simulink model "part2_MAIN_2019_for_ayon_because_he_cant_update_his_matlab"  (R2019a)
settings: Solver=FixedStepAuto  StartTime=0.0  StopTime=300  FixedStep=0.1  RelTol=1e-3
values from neighbouring files (symbols this model uses):
  Af = diag(ti)    [init.m]    (also in init_old.m)
  Aw = [zeros(3) eye(3) ... (first row only)    [get_observer_parameters.m]
  B = [thr1 thr2_x thr2_y thr3 thr4_x thr4_y thr5_x thr5_y]    [B_redistributed.m]    (also in check_alg.m = [1 2 3 4 5 6 7 8; get_observer_parameters.m = [zeros(6,3);zeros(3,3);zeros(3,3);inv(M)])
  change_position_time = 1200    [init.m]    (also in init_old.m)
  Cw = [zeros(3) eye(3)]    [get_observer_parameters.m]
  D = Damping    [init.m]    (also in init_old.m)
  Damping = diag([2.6486e5, 8.8164e5, 3.3774e8])    [init.m]    (also in init_old.m)
  direction_limit = pi/36    (= 0.0872664625997)    [init.m]    (also in init_old.m)
  direction_time_constant = 100    [init.m]    (also in init_old.m)
  dt = 0.1    [get_observer_parameters.m]
  E = [Ew, zeros(6,3) ... (first row only)    [get_observer_parameters.m]
  Gamma = diag(omega_is)    [init.m]    (also in init_old.m)
  gust_limit = 40    [init.m]    (also in init_old.m)
  H = [Cw, eye(3), zeros(3,3) zeros(3,3)]    [get_observer_parameters.m]    (also in quadprog.m = 2*diag([w.' w.' q.' q.' w_alpha.' w_alpha.']); quadprog_basic.m = 2*diag([w.' w.' q.' q.']); quadprog_false.m = 2*diag([w.' w.' q.' q.' w_alpha.' w_alpha.']))
  height = 3    [init.m]    (also in init_old.m)
  inv_M = inv(M)    [get_observer_parameters.m]
  inv_Tb = inv(Tb)    [get_observer_parameters.m]
  kappa = 0.003    [init.m]    (also in init_old.m)
  kappa2 = 0.0026    [init.m]    (also in init_old.m)
  Kd = [1660451.40544401; 3920391.80535684; 1605063439.04156]    [init.m]    (also in init_old.m)
  Ki = [137.081306245593; 3163.274947400198; 335358.448218978]    [init.m]    (also in init_old.m)
  Kp = [75459.3345349083; 277551.73586971; 120744473.878042]    [init.m]    (also in init_old.m)
  L = 1800    [init.m]    (also in init_old.m)
  M = Mass    [init.m]    (also in init_old.m)
  mean_wind_direction = pi    (= 3.14159265359)    [init.m]    (also in init_old.m)
  observer_type = 0    [init.m]    (also in init_old.m)
  Omega = diag([omega_n, omega_n, omega_n])    [get_observer_parameters.m]    (also in init.m = diag(2*omega_is.*zeta_is); init_old.m = diag(2*omega_is.*zeta_is))
  Q = diag([0.1,0.1,pi/180,1e6,1e6,1e9])*10e3    [get_observer_parameters.m]
  R = diag([1,0.1,0.1*pi/180])*10e-3    [get_observer_parameters.m]
  simulation = 7    [init.m]    (also in init_old.m = 1)
  slow_varying_limit = 1    [init.m]    (also in init_old.m)
  slow_varying_time_constant = 100    [init.m]    (also in init_old.m)
  TAU = dt*E    [get_observer_parameters.m]
  Tb = 0.1 * eye(3)    [get_observer_parameters.m]
  thruster_type = 0    [init.m]    (also in init_old.m)
  u10 = 12    [init.m]    (also in init_old.m)
  vessel =     [test.mat]
  wind = 1    [init.m]    (also in init_old.m)
undefined symbols (not defined in the file or in its folder): Hoerner, ModelParams, npf, Param, thrusters, WaveModel
libraries: simulink x49, dspsigops x39, marine_hydro x14, marine_gnc x7
(part 1 of 9)
settings Model: Creator=jonbjor  LastModifiedBy=aduragbemi
settings DataIOCC: ReturnWorkspaceOutputs=off
settings DebuggingCC: ArithmeticOperatorsInVariantConditions=warning
settings SFSimCC: SimUseLocalCustomCode=off
settings RTWCC: RTWUseLocalCustomCode=off

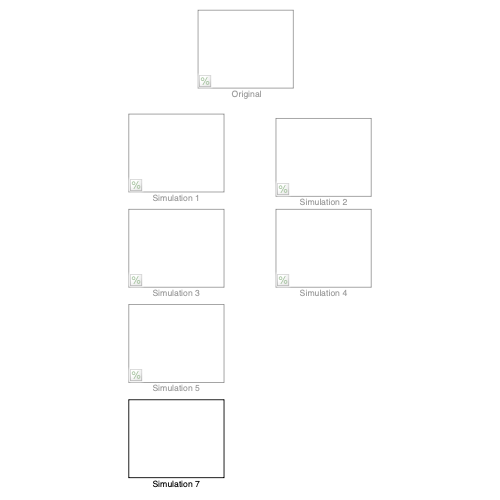
[thumbnail: Simulink's stored preview of the top-level diagram]
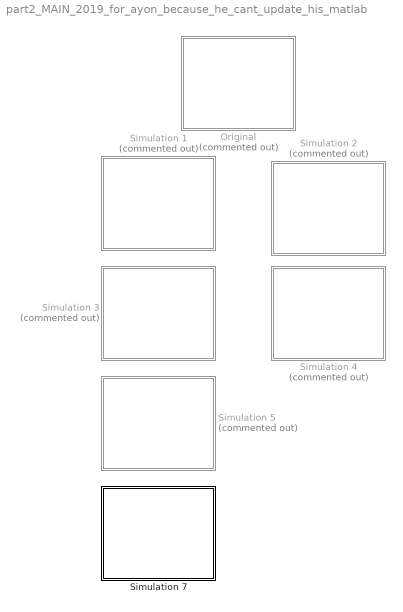
== system part2_MAIN_2019_for_ayon_because_he_cant_update_his_matlab ==
  " Original" : Subsystem  Commented=on
  Simulation 1 : Subsystem  Commented=on
  Simulation 2 : Subsystem  Commented=on
  Simulation 3 : Subsystem  Commented=on
  Simulation 4 : Subsystem  Commented=on
  Simulation 5 : Subsystem  Commented=on
  Simulation 7 : Subsystem

== system part2_MAIN_2019_for_ayon_because_he_cant_update_his_matlab/ Original ==
  Current (North - East) : Subsystem
  DP Controller : Subsystem
  Observer : Subsystem
  Reference Model : Subsystem
  Scope : Scope  NumInputPorts=2
  Scope1 : Scope  NumInputPorts=2
  Scope2 : Scope  NumInputPorts=2
  Selector : Selector  InputPortWidth=6  IndexOptions=Index vector (dialog)  Indices=[1 2 6]  OutputSizes=1
  Selector1 : Selector  InputPortWidth=6  IndexOptions=Index vector (dialog)  Indices=[1 2 6]  OutputSizes=1
  Service Operation Vessel - SOV : marine_hydro/Hydro Library/6 DOF DP model  (zero speed model with fluid memory)  ABC=vesselABC  rho=1025  Axc=0.9*vessel.main.T*vessel.main.B  Ayc=0.9*vessel.main.T*vessel.main.Lpp  CX=1  CY_2D=Hoerner(vessel.main.B,vessel.main.T)  Bv=vessel.Bv  mask(6 DOF zero speed model){}
      link override "Integrator1 ": InitialCondition=nu0
      link override Integrator2: InitialCondition=eta0
      mask Display:
      | image('SOV.jpg');
      | color('white'); port_label('output', 1, 'eta')
      | color('white'); port_label('output', 2, 'nu')
      | color('white'); port_label('input', 1, 'tau_wave')
      | color('white'); port_label('input', 2, 'tau')
      | color('white'); port_label('input', 3, 'nu_c')
  Sum : Sum  Inputs=|++
  Terminator : Terminator
  Terminator1 : Terminator
  Thrust Allocation : Subsystem
  Thruster Dynamics : Subsystem  mask{thrusterfault=off}
      mask prompts: thrusterfault "Fault on thruster #2 and #4?"
  To Workspace : ToWorkspace  VariableName=Eta_obs  SaveFormat=Timeseries  SampleTime=-1
  To Workspace1 : ToWorkspace  VariableName=Eta  SaveFormat=Timeseries  SampleTime=-1
  To Workspace2 : ToWorkspace  VariableName=nu  SaveFormat=Timeseries  SampleTime=-1
  To Workspace3 : ToWorkspace  VariableName=nu_obs  SaveFormat=Timeseries  SampleTime=-1
  To Workspace4 : ToWorkspace  VariableName=nu_sp  SaveFormat=Timeseries  SampleTime=-1
  To Workspace5 : ToWorkspace  VariableName=Eta_sp  SaveFormat=Timeseries  SampleTime=-1
  Wave : Subsystem  mask{waveforces=on}
      mask prompts: waveforces "Waveforces enabled"
  Waves : marine_gnc/Environment/Waves/Waves  spectrum_type=ITTC  disp_flag=on  plot_spectrum=off  plot_realization=off  hs=2.5  omega_peak=2*pi/9  psi_mean=-3*pi/4  gamma=-1  spread=2  depth=inf  nfreq=20  ndir=10  energylim=0.005  freq_cutoff=3  dir_cutoff=0  rand_seed=123  rand_freq=on  rand_dir=on  Zeta_a=0  Omega=0  Phase=0  Wavenum=0  Psi=0
  Wind : Subsystem
  wires:
  Waves/1 -> Wave/2(waves)
  Selector/1 -> Wind/1(eta), Scope/1, To Workspace1/1, Observer/1(y), Current (North - East)/1(eta)  "eta"
  Sum/1 -> Service Operation Vessel - SOV/2
  Thruster Dynamics/1("Forces (body frame) ") -> Scope2/2, Sum/1
  Observer/1(nu_hat) -> To Workspace3/1, Scope1/2, DP Controller/1(nu)
  Service Operation Vessel - SOV/2 -> Selector1/1
  Wind/1(Wind) -> Sum/2
  Wave/1(Wave) -> Service Operation Vessel - SOV/1
  DP Controller/1(tau (body frame)) -> Scope2/1, Observer/2(tau_est)
  Reference Model/2(nu set point) -> To Workspace4/1, DP Controller/4(nu setpoint)
  Waves/2 -> Terminator/1
  Observer/2(eta_hat) -> DP Controller/2(eta), Scope/2, To Workspace/1
  Thrust Allocation/1(u) -> Thruster Dynamics/1(u [N])
  Reference Model/1(Set-point) -> DP Controller/3(eta set point), To Workspace5/1
  Service Operation Vessel - SOV/1 -> Wave/1(eta), Selector/1
  Thrust Allocation/2(alpha [rad]) -> Thruster Dynamics/2(alpha [rad])
  Current (North - East)/1(Current1) -> Service Operation Vessel - SOV/3
  Selector1/1 -> Wind/2(nu), To Workspace2/1, Scope1/1, Terminator1/1

== system part2_MAIN_2019_for_ayon_because_he_cant_update_his_matlab/Simulation 1 ==
  Controller_force : ToWorkspace  VariableName=Controller_force  SaveFormat=Timeseries  SampleTime=-1
  Current (North - East) : Subsystem
  DP Controller : Subsystem
  Demux : Demux  Outputs=3
  Gain : Gain  Gain=180/pi
  Observer : Subsystem  Commented=on
  Reference Model : Subsystem
  Scope : Scope  NumInputPorts=3
  Scope1 : Scope  NumInputPorts=2
  Scope2 : Scope  NumInputPorts=3
  Scope3 : Scope  NumInputPorts=3
  Selector : Selector  InputPortWidth=6  IndexOptions=Index vector (dialog)  Indices=[1 2 6]  OutputSizes=1
  Selector1 : Selector  InputPortWidth=6  IndexOptions=Index vector (dialog)  Indices=[1 2 6]  OutputSizes=1
  Service Operation Vessel - SOV : marine_hydro/Hydro Library/6 DOF DP model  (zero speed model with fluid memory)  ABC=vesselABC  rho=1025  Axc=0.9*vessel.main.T*vessel.main.B  Ayc=0.9*vessel.main.T*vessel.main.Lpp  CX=1  CY_2D=Hoerner(vessel.main.B,vessel.main.T)  Bv=vessel.Bv  mask(6 DOF zero speed model){}
      link override "Integrator1 ": InitialCondition=nu0
      link override Integrator2: InitialCondition=eta0
      mask Display:
      | image('SOV.jpg');
      | color('white'); port_label('output', 1, 'eta')
      | color('white'); port_label('output', 2, 'nu')
      | color('white'); port_label('input', 1, 'tau_wave')
      | color('white'); port_label('input', 2, 'tau')
      | color('white'); port_label('input', 3, 'nu_c')
  Sum : Sum  Inputs=|++
  Terminator : Terminator
  Terminator1 : Terminator
  Thrust Allocation : Subsystem
  Thrust_dynamic_force : ToWorkspace  VariableName=Thrust_dynamic_force  SaveFormat=Timeseries  SampleTime=-1
  Thruster Dynamics : Subsystem  mask{thrusterfault=on}
      mask prompts: thrusterfault "Fault on thruster #2 and #4?"
  Thruster_force : ToWorkspace  Commented=on  VariableName=Thruster_force  SaveFormat=Timeseries  SampleTime=-1
  To Workspace : ToWorkspace  Commented=on  VariableName=Eta_obs  SaveFormat=Timeseries  SampleTime=-1
  To Workspace1 : ToWorkspace  VariableName=Eta  SaveFormat=Timeseries  SampleTime=-1
  To Workspace2 : ToWorkspace  VariableName=nu  SaveFormat=Timeseries  SampleTime=-1
  To Workspace3 : ToWorkspace  Commented=on  VariableName=nu_obs  SaveFormat=Timeseries  SampleTime=-1
  To Workspace4 : ToWorkspace  VariableName=nu_sp  SaveFormat=Timeseries  SampleTime=-1
  To Workspace5 : ToWorkspace  VariableName=Eta_sp  SaveFormat=Timeseries  SampleTime=-1
  Wave : Subsystem  mask{waveforces=on}
      mask prompts: waveforces "Waveforces enabled"
  Waves : marine_gnc/Environment/Waves/Waves  spectrum_type=ITTC  disp_flag=on  plot_spectrum=off  plot_realization=off  hs=2.5  omega_peak=2*pi/9  psi_mean=-3*pi/4  gamma=-1  spread=2  depth=inf  nfreq=20  ndir=10  energylim=0.005  freq_cutoff=3  dir_cutoff=0  rand_seed=123  rand_freq=on  rand_dir=on  Zeta_a=0  Omega=0  Phase=0  Wavenum=0  Psi=0
  Wind : Subsystem
  wires:
  Waves/1 -> Wave/2(waves)
  Selector/1 -> Wind/1(eta), DP Controller/2(eta), Scope/1, Demux/1, To Workspace1/1, Observer/1(y), Current (North - East)/1(eta)  "eta"
  Sum/1 -> Service Operation Vessel - SOV/2
  Thruster Dynamics/1("Forces (body frame) ") -> Scope2/2, Thrust_dynamic_force/1
  Observer/1(nu_hat) -> To Workspace3/1
  Service Operation Vessel - SOV/2 -> Selector1/1
  Wind/1(Wind) -> Sum/2
  Wave/1(Wave) -> Service Operation Vessel - SOV/1
  DP Controller/1(tau (body frame)) -> Scope2/1, Thrust Allocation/1(tau_d), Controller_force/1, Observer/2(tau_est)
  Reference Model/2(nu set point) -> To Workspace4/1, Scope1/2, DP Controller/4(nu setpoint)
  Waves/2 -> Terminator/1
  Observer/2(eta_hat) -> Scope/2, To Workspace/1
  Thrust Allocation/1(u) -> Scope2/3, Thruster_force/1, Thruster Dynamics/1(u [N])
  Reference Model/1(Set-point) -> DP Controller/3(eta set point), To Workspace5/1, Scope/3
  Service Operation Vessel - SOV/1 -> Wave/1(eta), Selector/1
  Thrust Allocation/2(alpha [rad]) -> Thruster Dynamics/2(alpha [rad])
  Current (North - East)/1(Current1) -> Service Operation Vessel - SOV/3
  Selector1/1 -> Wind/2(nu), DP Controller/1(nu), To Workspace2/1, Scope1/1, Terminator1/1
  Demux/3 -> Gain/1
  Gain/1 -> Scope3/3
  Demux/1 -> Scope3/1
  Demux/2 -> Scope3/2

== system part2_MAIN_2019_for_ayon_because_he_cant_update_his_matlab/Simulation 2 ==
  Controller_force : ToWorkspace  VariableName=Controller_force  SaveFormat=Timeseries  SampleTime=-1
  Current (North - East) : Subsystem  Commented=on
  DP Controller : Subsystem
  Observer : Subsystem  Commented=on
  Reference Model : Subsystem
  Scope : Scope  NumInputPorts=3
  Scope1 : Scope  NumInputPorts=2
  Scope2 : Scope  NumInputPorts=3
  Selector : Selector  InputPortWidth=6  IndexOptions=Index vector (dialog)  Indices=[1 2 6]  OutputSizes=1
  Selector1 : Selector  InputPortWidth=6  IndexOptions=Index vector (dialog)  Indices=[1 2 6]  OutputSizes=1
  Service Operation Vessel - SOV : marine_hydro/Hydro Library/6 DOF DP model  (zero speed model with fluid memory)  ABC=vesselABC  rho=1025  Axc=0.9*vessel.main.T*vessel.main.B  Ayc=0.9*vessel.main.T*vessel.main.Lpp  CX=1  CY_2D=Hoerner(vessel.main.B,vessel.main.T)  Bv=vessel.Bv  mask(6 DOF zero speed model){}
      link override "Integrator1 ": InitialCondition=nu0
      link override Integrator2: InitialCondition=eta0
      mask Display:
      | image('SOV.jpg');
      | color('white'); port_label('output', 1, 'eta')
      | color('white'); port_label('output', 2, 'nu')
      | color('white'); port_label('input', 1, 'tau_wave')
      | color('white'); port_label('input', 2, 'tau')
      | color('white'); port_label('input', 3, 'nu_c')
  Sum : Sum  Inputs=|++
  Terminator : Terminator
  Terminator1 : Terminator
  Thrust Allocation : Subsystem
  Thrust_dynamic_force : ToWorkspace  VariableName=Thrust_dynamic_force  SaveFormat=Timeseries  SampleTime=-1
  Thruster Dynamics : Subsystem  mask{thrusterfault=on}
      mask prompts: thrusterfault "Fault on thruster #2 and #4?"
  Thruster_force : ToWorkspace  Commented=on  VariableName=Thruster_force  SaveFormat=Timeseries  SampleTime=-1
  To Workspace : ToWorkspace  Commented=on  VariableName=Eta_obs  SaveFormat=Timeseries  SampleTime=-1
  To Workspace1 : ToWorkspace  VariableName=Eta  SaveFormat=Timeseries  SampleTime=-1
  To Workspace2 : ToWorkspace  VariableName=nu  SaveFormat=Timeseries  SampleTime=-1
  To Workspace3 : ToWorkspace  Commented=on  VariableName=nu_obs  SaveFormat=Timeseries  SampleTime=-1
  To Workspace4 : ToWorkspace  VariableName=nu_sp  SaveFormat=Timeseries  SampleTime=-1
  To Workspace5 : ToWorkspace  VariableName=Eta_sp  SaveFormat=Timeseries  SampleTime=-1
  Wave : Subsystem  Commented=on  mask{waveforces=off}
      mask prompts: waveforces "Waveforces enabled"
  Waves : marine_gnc/Environment/Waves/Waves  spectrum_type=ITTC  disp_flag=on  plot_spectrum=off  plot_realization=off  hs=2.5  omega_peak=2*pi/9  psi_mean=-3*pi/4  gamma=-1  spread=2  depth=inf  nfreq=20  ndir=10  energylim=0.005  freq_cutoff=3  dir_cutoff=0  rand_seed=123  rand_freq=on  rand_dir=on  Zeta_a=0  Omega=0  Phase=0  Wavenum=0  Psi=0
  Wind : Subsystem  Commented=on
  wires:
  Waves/1 -> Wave/2(waves)
  Selector/1 -> Wind/1(eta), DP Controller/2(eta), Scope/1, To Workspace1/1, Observer/1(y), Current (North - East)/1(eta)  "eta"
  Sum/1 -> Service Operation Vessel - SOV/2
  Thruster Dynamics/1("Forces (body frame) ") -> Sum/1, Scope2/2, Thrust_dynamic_force/1
  Observer/1(nu_hat) -> To Workspace3/1
  Service Operation Vessel - SOV/2 -> Selector1/1
  Wind/1(Wind) -> Sum/2
  Wave/1(Wave) -> Service Operation Vessel - SOV/1
  DP Controller/1(tau (body frame)) -> Scope2/1, Thrust Allocation/1(tau_d), Controller_force/1, Observer/2(tau_est)
  Reference Model/2(nu set point) -> To Workspace4/1, Scope1/2, DP Controller/4(nu setpoint)
  Waves/2 -> Terminator/1
  Observer/2(eta_hat) -> Scope/2, To Workspace/1
  Thrust Allocation/1(u) -> Scope2/3, Thruster_force/1, Thruster Dynamics/1(u [N])
  Reference Model/1(Set-point) -> DP Controller/3(eta set point), To Workspace5/1, Scope/3
  Service Operation Vessel - SOV/1 -> Wave/1(eta), Selector/1
  Thrust Allocation/2(alpha [rad]) -> Thruster Dynamics/2(alpha [rad])
  Current (North - East)/1(Current1) -> Service Operation Vessel - SOV/3
  Selector1/1 -> Wind/2(nu), DP Controller/1(nu), To Workspace2/1, Scope1/1, Terminator1/1

== system part2_MAIN_2019_for_ayon_because_he_cant_update_his_matlab/Simulation 3 ==
  Controller_force : ToWorkspace  VariableName=Controller_force  SaveFormat=Timeseries  SampleTime=-1
  Current (North - East) : Subsystem
  DP Controller : Subsystem
  Observer : Subsystem  Commented=on
  Reference Model : Subsystem
  Scope : Scope  NumInputPorts=3
  Scope1 : Scope  NumInputPorts=2
  Scope2 : Scope  NumInputPorts=3
  Selector : Selector  InputPortWidth=6  IndexOptions=Index vector (dialog)  Indices=[1 2 6]  OutputSizes=1
  Selector1 : Selector  InputPortWidth=6  IndexOptions=Index vector (dialog)  Indices=[1 2 6]  OutputSizes=1
  Service Operation Vessel - SOV : marine_hydro/Hydro Library/6 DOF DP model  (zero speed model with fluid memory)  ABC=vesselABC  rho=1025  Axc=0.9*vessel.main.T*vessel.main.B  Ayc=0.9*vessel.main.T*vessel.main.Lpp  CX=1  CY_2D=Hoerner(vessel.main.B,vessel.main.T)  Bv=vessel.Bv  mask(6 DOF zero speed model){}
      link override "Integrator1 ": InitialCondition=nu0
      link override Integrator2: InitialCondition=eta0
      mask Display:
      | image('SOV.jpg');
      | color('white'); port_label('output', 1, 'eta')
      | color('white'); port_label('output', 2, 'nu')
      | color('white'); port_label('input', 1, 'tau_wave')
      | color('white'); port_label('input', 2, 'tau')
      | color('white'); port_label('input', 3, 'nu_c')
  Sum : Sum  Inputs=|++
  Terminator : Terminator
  Terminator1 : Terminator
  Thrust Allocation : Subsystem
  Thrust_dynamic_force : ToWorkspace  VariableName=Thrust_dynamic_force  SaveFormat=Timeseries  SampleTime=-1
  Thruster Dynamics : Subsystem  mask{thrusterfault=off}
      mask prompts: thrusterfault "Fault on thruster #2 and #4?"
  Thruster_force : ToWorkspace  VariableName=Thruster_force  SaveFormat=Timeseries  SampleTime=-1
  To Workspace : ToWorkspace  Commented=on  VariableName=Eta_obs  SaveFormat=Timeseries  SampleTime=-1
  To Workspace1 : ToWorkspace  VariableName=Eta  SaveFormat=Timeseries  SampleTime=-1
  To Workspace2 : ToWorkspace  VariableName=nu  SaveFormat=Timeseries  SampleTime=-1
  To Workspace3 : ToWorkspace  Commented=on  VariableName=nu_obs  SaveFormat=Timeseries  SampleTime=-1
  To Workspace4 : ToWorkspace  VariableName=nu_sp  SaveFormat=Timeseries  SampleTime=-1
  To Workspace5 : ToWorkspace  VariableName=Eta_sp  SaveFormat=Timeseries  SampleTime=-1
  Wave : Subsystem  mask{waveforces=on}
      mask prompts: waveforces "Waveforces enabled"
  Waves : marine_gnc/Environment/Waves/Waves  spectrum_type=ITTC  disp_flag=on  plot_spectrum=off  plot_realization=off  hs=2.5  omega_peak=2*pi/9  psi_mean=-3*pi/4  gamma=-1  spread=2  depth=inf  nfreq=20  ndir=10  energylim=0.005  freq_cutoff=3  dir_cutoff=0  rand_seed=123  rand_freq=on  rand_dir=on  Zeta_a=0  Omega=0  Phase=0  Wavenum=0  Psi=0
  Wind : Subsystem
  wires:
  Waves/1 -> Wave/2(waves)
  Selector/1 -> Wind/1(eta), DP Controller/2(eta), Scope/1, To Workspace1/1, Observer/1(y), Current (North - East)/1(eta)  "eta"
  Sum/1 -> Service Operation Vessel - SOV/2
  Thruster Dynamics/1("Forces (body frame) ") -> Sum/1, Scope2/2, Thrust_dynamic_force/1
  Observer/1(nu_hat) -> To Workspace3/1
  Service Operation Vessel - SOV/2 -> Selector1/1
  Wind/1(Wind) -> Sum/2
  Wave/1(Wave) -> Service Operation Vessel - SOV/1
  DP Controller/1(tau (body frame)) -> Scope2/1, Thrust Allocation/1(tau_d), Controller_force/1, Observer/2(tau_est)
  Reference Model/2(nu set point) -> To Workspace4/1, Scope1/2, DP Controller/4(nu setpoint)
  Waves/2 -> Terminator/1
  Observer/2(eta_hat) -> Scope/2, To Workspace/1
  Thrust Allocation/1(u) -> Scope2/3, Thruster_force/1, Thruster Dynamics/1(u [N])
  Reference Model/1(Set-point) -> DP Controller/3(eta set point), To Workspace5/1, Scope/3
  Service Operation Vessel - SOV/1 -> Wave/1(eta), Selector/1
  Thrust Allocation/2(alpha [rad]) -> Thruster Dynamics/2(alpha [rad])
  Current (North - East)/1(Current1) -> Service Operation Vessel - SOV/3
  Selector1/1 -> Wind/2(nu), DP Controller/1(nu), To Workspace2/1, Scope1/1, Terminator1/1

== system part2_MAIN_2019_for_ayon_because_he_cant_update_his_matlab/Simulation 4 ==
  Constant : Constant  Value=[1;1;0;0;0;1]*10^4
  Controller_force : ToWorkspace  Commented=on  VariableName=Controller_force  SaveFormat=Timeseries  SampleTime=-1
  Current (North - East) : Subsystem
  DP Controller : Subsystem
  Observer : Subsystem
  Reference Model : Subsystem
  Scope : Scope  NumInputPorts=3
  Scope1 : Scope  NumInputPorts=2
  Scope2 : Scope  NumInputPorts=3
  Selector : Selector  InputPortWidth=6  IndexOptions=Index vector (dialog)  Indices=[1 2 6]  OutputSizes=1
  Selector1 : Selector  InputPortWidth=6  IndexOptions=Index vector (dialog)  Indices=[1 2 6]  OutputSizes=1
  Service Operation Vessel - SOV : marine_hydro/Hydro Library/6 DOF DP model  (zero speed model with fluid memory)  ABC=vesselABC  rho=1025  Axc=0.9*vessel.main.T*vessel.main.B  Ayc=0.9*vessel.main.T*vessel.main.Lpp  CX=1  CY_2D=Hoerner(vessel.main.B,vessel.main.T)  Bv=vessel.Bv  mask(6 DOF zero speed model){}
      link override "Integrator1 ": InitialCondition=nu0
      link override Integrator2: InitialCondition=eta0
      mask Display:
      | image('SOV.jpg');
      | color('white'); port_label('output', 1, 'eta')
      | color('white'); port_label('output', 2, 'nu')
      | color('white'); port_label('input', 1, 'tau_wave')
      | color('white'); port_label('input', 2, 'tau')
      | color('white'); port_label('input', 3, 'nu_c')
  Sum : Sum  Inputs=|++
  Terminator : Terminator
  Terminator1 : Terminator
  Thrust Allocation : Subsystem
  Thrust_dynamic_force : ToWorkspace  VariableName=Thrust_dynamic_force  SaveFormat=Timeseries  SampleTime=-1
  Thruster Dynamics : Subsystem  mask{thrusterfault=off}
      mask prompts: thrusterfault "Fault on thruster #2 and #4?"
  Thruster_force : ToWorkspace  VariableName=Thruster_force  SaveFormat=Timeseries  SampleTime=-1
  To Workspace : ToWorkspace  VariableName=Eta_obs  SaveFormat=Timeseries  SampleTime=-1
  To Workspace1 : ToWorkspace  VariableName=Eta  SaveFormat=Timeseries  SampleTime=-1
  To Workspace2 : ToWorkspace  VariableName=nu  SaveFormat=Timeseries  SampleTime=-1
  To Workspace3 : ToWorkspace  VariableName=nu_obs  SaveFormat=Timeseries  SampleTime=-1
  To Workspace4 : ToWorkspace  VariableName=nu_sp  SaveFormat=Timeseries  SampleTime=-1
  To Workspace5 : ToWorkspace  VariableName=Eta_sp  SaveFormat=Timeseries  SampleTime=-1
  Wave : Subsystem  mask{waveforces=on}
      mask prompts: waveforces "Waveforces enabled"
  Waves : marine_gnc/Environment/Waves/Waves  spectrum_type=ITTC  disp_flag=on  plot_spectrum=off  plot_realization=off  hs=2.5  omega_peak=2*pi/9  psi_mean=-3*pi/4  gamma=-1  spread=2  depth=inf  nfreq=20  ndir=10  energylim=0.005  freq_cutoff=3  dir_cutoff=0  rand_seed=123  rand_freq=on  rand_dir=on  Zeta_a=0  Omega=0  Phase=0  Wavenum=0  Psi=0
  Wind : Subsystem
  wires:
  Constant/1 -> Observer/2(tau_est), Thrust Allocation/1(tau_d)
  Waves/1 -> Wave/2(waves)
  Selector/1 -> Wind/1(eta), Scope/1, To Workspace1/1, Observer/1(y), Current (North - East)/1(eta)  "eta"
  Sum/1 -> Service Operation Vessel - SOV/2
  Thruster Dynamics/1("Forces (body frame) ") -> Sum/1, Scope2/2, Thrust_dynamic_force/1
  Observer/1(nu_hat) -> To Workspace3/1, DP Controller/1(nu)
  Service Operation Vessel - SOV/2 -> Selector1/1
  Wind/1(Wind) -> Sum/2
  Wave/1(Wave) -> Service Operation Vessel - SOV/1
  DP Controller/1(tau (body frame)) -> Scope2/1
  Reference Model/2(nu set point) -> To Workspace4/1, Scope1/2, DP Controller/4(nu setpoint)
  Waves/2 -> Terminator/1
  Observer/2(eta_hat) -> To Workspace/1, Scope/2, DP Controller/2(eta)
  Thrust Allocation/1(u) -> Scope2/3, Thruster_force/1, Thruster Dynamics/1(u [N])
  Reference Model/1(Set-point) -> DP Controller/3(eta set point), To Workspace5/1, Scope/3
  Service Operation Vessel - SOV/1 -> Wave/1(eta), Selector/1
  Thrust Allocation/2(alpha [rad]) -> Thruster Dynamics/2(alpha [rad])
  Current (North - East)/1(Current1) -> Service Operation Vessel - SOV/3
  Selector1/1 -> Wind/2(nu), To Workspace2/1, Scope1/1, Terminator1/1

== system part2_MAIN_2019_for_ayon_because_he_cant_update_his_matlab/Simulation 5 ==
  Controller_force : ToWorkspace  VariableName=Controller_force  SaveFormat=Timeseries  SampleTime=-1
  Current (North - East) : Subsystem
  DP Controller : Subsystem
  Observer : Subsystem
  Reference Model : Subsystem
  Scope : Scope  NumInputPorts=3
  Scope1 : Scope  NumInputPorts=2
  Scope2 : Scope  NumInputPorts=2
  Selector : Selector  InputPortWidth=6  IndexOptions=Index vector (dialog)  Indices=[1 2 6]  OutputSizes=1
  Selector1 : Selector  InputPortWidth=6  IndexOptions=Index vector (dialog)  Indices=[1 2 6]  OutputSizes=1
  Service Operation Vessel - SOV : marine_hydro/Hydro Library/6 DOF DP model  (zero speed model with fluid memory)  ABC=vesselABC  rho=1025  Axc=0.9*vessel.main.T*vessel.main.B  Ayc=0.9*vessel.main.T*vessel.main.Lpp  CX=1  CY_2D=Hoerner(vessel.main.B,vessel.main.T)  Bv=vessel.Bv  mask(6 DOF zero speed model){}
      link override "Integrator1 ": InitialCondition=nu0
      link override Integrator2: InitialCondition=eta0
      mask Display:
      | image('SOV.jpg');
      | color('white'); port_label('output', 1, 'eta')
      | color('white'); port_label('output', 2, 'nu')
      | color('white'); port_label('input', 1, 'tau_wave')
      | color('white'); port_label('input', 2, 'tau')
      | color('white'); port_label('input', 3, 'nu_c')
  Sum : Sum  Inputs=|++
  Terminator : Terminator
  Terminator1 : Terminator
  Thrust Allocation : Subsystem
  Thrust_dynamic_force : ToWorkspace  VariableName=Thrust_dynamic_force1  SaveFormat=Timeseries  SampleTime=-1
  Thruster Dynamics : Subsystem  mask{thrusterfault=off}
      mask prompts: thrusterfault "Fault on thruster #2 and #4?"
  Thruster_force : ToWorkspace  VariableName=Thruster_force  SaveFormat=Timeseries  SampleTime=-1
  To Workspace : ToWorkspace  VariableName=Eta_obs  SaveFormat=Timeseries  SampleTime=-1
  To Workspace1 : ToWorkspace  VariableName=Eta  SaveFormat=Timeseries  SampleTime=-1
  To Workspace2 : ToWorkspace  VariableName=nu  SaveFormat=Timeseries  SampleTime=-1
  To Workspace3 : ToWorkspace  VariableName=nu_obs  SaveFormat=Timeseries  SampleTime=-1
  To Workspace4 : ToWorkspace  VariableName=nu_sp  SaveFormat=Timeseries  SampleTime=-1
  To Workspace5 : ToWorkspace  VariableName=Eta_sp  SaveFormat=Timeseries  SampleTime=-1
  Wave : Subsystem  mask{waveforces=on}
      mask prompts: waveforces "Waveforces enabled"
  Waves : marine_gnc/Environment/Waves/Waves  spectrum_type=ITTC  disp_flag=on  plot_spectrum=off  plot_realization=off  hs=2.5  omega_peak=2*pi/9  psi_mean=-3*pi/4  gamma=-1  spread=2  depth=inf  nfreq=20  ndir=10  energylim=0.005  freq_cutoff=3  dir_cutoff=0  rand_seed=123  rand_freq=on  rand_dir=on  Zeta_a=0  Omega=0  Phase=0  Wavenum=0  Psi=0
  Wind : Subsystem
  wires:
  Waves/1 -> Wave/2(waves)
  Selector/1 -> Wind/1(eta), Scope/1, To Workspace1/1, Observer/1(y), Current (North - East)/1(eta)  "eta"
  Sum/1 -> Service Operation Vessel - SOV/2
  Thruster Dynamics/1("Forces (body frame) ") -> Sum/1, Scope2/2, Thrust_dynamic_force/1
  Observer/1(nu_hat) -> To Workspace3/1, Scope1/2, DP Controller/1(nu)
  Service Operation Vessel - SOV/2 -> Selector1/1
  Wind/1(Wind) -> Sum/2
  Wave/1(Wave) -> Service Operation Vessel - SOV/1
  DP Controller/1(tau (body frame)) -> Scope2/1, Controller_force/1, Observer/2(tau_est), Thrust Allocation/1(tau_d)
  Reference Model/2(nu set point) -> To Workspace4/1, DP Controller/4(nu setpoint)
  Waves/2 -> Terminator/1
  Observer/2(eta_hat) -> DP Controller/2(eta), Scope/2, To Workspace/1
  Thrust Allocation/1(u) -> Thruster_force/1, Thruster Dynamics/1(u [N])
  Reference Model/1(Set-point) -> DP Controller/3(eta set point), To Workspace5/1, Scope/3
  Service Operation Vessel - SOV/1 -> Wave/1(eta), Selector/1
  Thrust Allocation/2(alpha [rad]) -> Thruster Dynamics/2(alpha [rad])
  Current (North - East)/1(Current1) -> Service Operation Vessel - SOV/3
  Selector1/1 -> Wind/2(nu), To Workspace2/1, Scope1/1, Terminator1/1

== system part2_MAIN_2019_for_ayon_because_he_cant_update_his_matlab/Simulation 7 ==
  Controller_force : ToWorkspace  VariableName=Controller_force  SaveFormat=Timeseries  SampleTime=-1
  Current (North - East) : Subsystem
  DP Controller : Subsystem
  Observer : Subsystem
  Reference Model : Subsystem
  Scope : Scope  NumInputPorts=3
  Scope1 : Scope  NumInputPorts=2
  Scope2 : Scope  NumInputPorts=2
  Selector : Selector  InputPortWidth=6  IndexOptions=Index vector (dialog)  Indices=[1 2 6]  OutputSizes=1
  Selector1 : Selector  InputPortWidth=6  IndexOptions=Index vector (dialog)  Indices=[1 2 6]  OutputSizes=1
  Service Operation Vessel - SOV : marine_hydro/Hydro Library/6 DOF DP model  (zero speed model with fluid memory)  ABC=vesselABC  rho=1025  Axc=0.9*vessel.main.T*vessel.main.B  Ayc=0.9*vessel.main.T*vessel.main.Lpp  CX=1  CY_2D=Hoerner(vessel.main.B,vessel.main.T)  Bv=vessel.Bv  mask(6 DOF zero speed model){}
      link override "Integrator1 ": InitialCondition=nu0
      link override Integrator2: InitialCondition=eta0
      mask Display:
      | image('SOV.jpg');
      | color('white'); port_label('output', 1, 'eta')
      | color('white'); port_label('output', 2, 'nu')
      | color('white'); port_label('input', 1, 'tau_wave')
      | color('white'); port_label('input', 2, 'tau')
      | color('white'); port_label('input', 3, 'nu_c')
  Sum : Sum  Inputs=|++
  Terminator : Terminator
  Terminator1 : Terminator
  Thrust Allocation : Subsystem
  Thrust_dynamic_force : ToWorkspace  VariableName=Thrust_dynamic_force1  SaveFormat=Timeseries  SampleTime=-1
  Thruster Dynamics : Subsystem  mask{thrusterfault=off}
      mask prompts: thrusterfault "Fault on thruster #2 and #4?"
  Thruster_force : ToWorkspace  VariableName=Thruster_force  SaveFormat=Timeseries  SampleTime=-1
  To Workspace : ToWorkspace  VariableName=Eta_obs  SaveFormat=Timeseries  SampleTime=-1
  To Workspace1 : ToWorkspace  VariableName=Eta  SaveFormat=Timeseries  SampleTime=-1
  To Workspace2 : ToWorkspace  VariableName=nu  SaveFormat=Timeseries  SampleTime=-1
  To Workspace3 : ToWorkspace  VariableName=nu_obs  SaveFormat=Timeseries  SampleTime=-1
  To Workspace4 : ToWorkspace  VariableName=nu_sp  SaveFormat=Timeseries  SampleTime=-1
  To Workspace5 : ToWorkspace  VariableName=Eta_sp  SaveFormat=Timeseries  SampleTime=-1
  Wave : Subsystem  mask{waveforces=on}
      mask prompts: waveforces "Waveforces enabled"
  Waves : marine_gnc/Environment/Waves/Waves  spectrum_type=ITTC  disp_flag=on  plot_spectrum=off  plot_realization=off  hs=8  omega_peak=2*pi/13  psi_mean=-3*pi/4  gamma=-1  spread=2  depth=inf  nfreq=20  ndir=10  energylim=0.005  freq_cutoff=3  dir_cutoff=0  rand_seed=123  rand_freq=on  rand_dir=on  Zeta_a=0  Omega=0  Phase=0  Wavenum=0  Psi=0
  Wind : Subsystem
  wires:
  Waves/1 -> Wave/2(waves)
  Selector/1 -> Wind/1(eta), Scope/1, To Workspace1/1, Observer/1(y), Current (North - East)/1(eta)  "eta"
  Sum/1 -> Service Operation Vessel - SOV/2
  Thruster Dynamics/1("Forces (body frame) ") -> Sum/1, Scope2/2, Thrust_dynamic_force/1
  Observer/1(nu_hat) -> To Workspace3/1, Scope1/2, DP Controller/1(nu)
  Service Operation Vessel - SOV/2 -> Selector1/1
  Wind/1(Wind) -> Sum/2
  Wave/1(Wave) -> Service Operation Vessel - SOV/1
  DP Controller/1(tau (body frame)) -> Scope2/1, Controller_force/1, Observer/2(tau_est), Thrust Allocation/1(tau_d)
  Reference Model/2(nu set point) -> To Workspace4/1, DP Controller/4(nu setpoint)
  Waves/2 -> Terminator/1
  Observer/2(eta_hat) -> DP Controller/2(eta), Scope/2, To Workspace/1
  Thrust Allocation/1(u) -> Thruster_force/1, Thruster Dynamics/1(u [N])
  Reference Model/1(Set-point) -> DP Controller/3(eta set point), To Workspace5/1, Scope/3
  Service Operation Vessel - SOV/1 -> Wave/1(eta), Selector/1
  Thrust Allocation/2(alpha [rad]) -> Thruster Dynamics/2(alpha [rad])
  Current (North - East)/1(Current1) -> Service Operation Vessel - SOV/3
  Selector1/1 -> Wind/2(nu), To Workspace2/1, Scope1/1, Terminator1/1

== system part2_MAIN_2019_for_ayon_because_he_cant_update_his_matlab/ Original/Current (North - East) ==
  note: simulation 2
  note: simulation 1
  eta : Inport
  Constant : Constant  Value=simulation
  Constant1 : Constant  Value=[0.5*cos(135); 0.5*sin(135); 0]
  Demux : Demux  Outputs=3
  MATLAB Function : MATLAB Function  TreatAsAtomicUnit=on
  Matrix Multiply : Product  Multiplication=Matrix(*)
  Mux : Mux
  Scope : Scope  NumInputPorts=2
  Scope1 : Scope
  Step : Step  After=0  SampleTime=0
  Subsystem : Subsystem
  Subsystem1 : Subsystem
  Subsystem2 : Subsystem
  Switch : Switch  Criteria=u2 > Threshold  Threshold=1
  Switch1 : Switch  Criteria=u2 > Threshold  Threshold=2
  Terminator : Terminator
  Terminator1 : Terminator
  Terminator2 : Terminator
  To Workspace : ToWorkspace  VariableName=Current  SaveFormat=Timeseries  SampleTime=-1
  Current1 : Outport  VectorParamsAs1DForOutWhenUnconnected=off
  wires:
  Demux/2 -> Terminator1/1
  MATLAB Function/1(y) -> Matrix Multiply/1
  Switch/1 -> Switch1/3
  Matrix Multiply/1 -> Scope/2, Mux/1
  Subsystem2/1(Out1) -> Switch1/1
  Subsystem/1(Out1) -> Switch/3
  Subsystem1/1(Out1) -> Switch/1
  Demux/1 -> Terminator/1
  Switch1/1 -> Scope/1, To Workspace/1, Matrix Multiply/2
  eta/1 -> Demux/1  "eta"
  Constant/1 -> Switch1/2, Switch/2
  Constant1/1 -> Terminator2/1
  Step/1 -> Mux/3, Mux/2, Mux/4
  Demux/3 -> MATLAB Function/1(u)
  Mux/1 -> Scope1/1, Current1/1

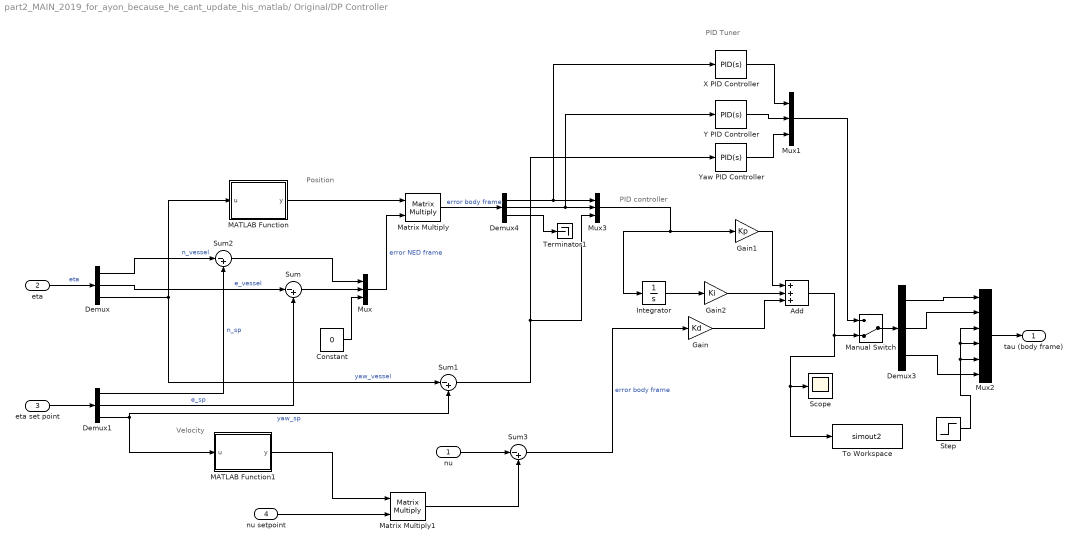
== system part2_MAIN_2019_for_ayon_because_he_cant_update_his_matlab/ Original/DP Controller ==
  note: PID Tuner
  note: PID controller
  note: Velocity
  note: Position
  nu : Inport
  eta : Inport  Port=2
  eta set point : Inport  Port=3
  nu setpoint : Inport  Port=4
  Add : Sum  Inputs=+++
  Constant : Constant  Value=0
  Demux{,1,3..4} (4 alike) : Demux  Outputs=3
  Gain : Gain  Gain=Kd
  Gain1 : Gain  Gain=Kp
  Gain2 : Gain  Gain=Ki
  Integrator : Integrator
  MATLAB Function : MATLAB Function  TreatAsAtomicUnit=on
  MATLAB Function1 : MATLAB Function  TreatAsAtomicUnit=on
  Manual Switch : ManualSwitch  CurrentSetting=0
  Matrix Multiply : Product  Multiplication=Matrix(*)
  Matrix Multiply1 : Product  Multiplication=Matrix(*)
  Mux : Mux  Inputs=3
  Mux1 : Mux  Inputs=3
  Mux2 : Mux  Inputs=6
  Mux3 : Mux  Inputs=3
  Scope : Scope
  Step : Step  After=0  SampleTime=0
  Sum{,1..3} (4 alike) : Sum  Inputs=|-+
  Terminator1 : Terminator
  To Workspace : ToWorkspace  VariableName=simout2  SaveFormat=Timeseries  SampleTime=-1
  X PID Controller : simulink/Continuous/PID Controller  Controller=PID  Form=Parallel  TimeDomain=Continuous-time  SampleTime=-1  IntegratorMethod=Forward Euler  FilterMethod=Forward Euler  ControllerParametersSource=internal  P=10219.9995649505  I=56.6576292157752  D=284184.955452018  N=0.143790431530358  UseFilter=on  TunerSelectOption=Transfer Function Based (PID Tuner App)  InitialConditionSource=internal  InitialConditionForIntegrator=0  InitialConditionForFilter=0  DifferentiatorICPrevScaledInput=0  ExternalReset=none  TrackingMode=off  Kt=1  LimitOutput=off  UpperSaturationLimit=inf  LowerSaturationLimit=-inf  LinearizeAsGain=on  AntiWindupMode=none  Kb=1  POutMin=[]  POutMax=[]  IOutMin=[]  IOutMax=[]  DOutMin=[]  DOutMax=[]  NOutMin=[]  NOutMax=[]  SumOutMin=[]  SumOutMax=[]  SaturationOutMin=[]  SaturationOutMax=[]  PParamMin=[]  PParamMax=[]  IParamMin=[]  IParamMax=[]  DParamMin=[]  DParamMax=[]  NParamMin=[]  NParamMax=[]  KbParamMin=[]  KbParamMax=[]  KtParamMin=[]  KtParamMax=[]  KbOutMin=[]  KbOutMax=[]  KtOutMin=[]  KtOutMax=[]  IntegratorOutMin=[]  IntegratorOutMax=[]  FilterOutMin=[]  FilterOutMax=[]  SumI1OutMin=[]  SumI1OutMax=[]  SumI2OutMin=[]  SumI2OutMax=[]  SumI3OutMin=[]  SumI3OutMax=[]  SumI4OutMin=[]  SumI4OutMax=[]  SumDOutMin=[]  SumDOutMax=[]  DifferentiatorOutMin=[]  DifferentiatorOutMax=[]  FilterDiffOutCoefMin=[]  FilterDiffOutCoefMax=[]  ReciprocalOutMin=[]  ReciprocalOutMax=[]  SumDenOutMin=[]  SumDenOutMax=[]  SumNumOutMin=[]  SumNumOutMax=[]  DivideOutMin=[]  DivideOutMax=[]  IntegratorContinuousStateAttributes=''  IntegratorStateMustResolveToSignalObject=off  IntegratorRTWStateStorageClass=Auto  FilterContinuousStateAttributes=''  FilterStateMustResolveToSignalObject=off  FilterRTWStateStorageClass=Auto  ParallelPVariant=InternalParameters  IdealPVariant=Disabled  IVariant=InternalParameters  DVariant=InternalParameters  IntegratorVariant=Continuous  SatVariant=Disabled  AWVariant=Passthrough  PCopyVariant=Disabled  TRVariant=Disabled  FdbkBlocksVariant=Forward  IdealPFdbkVariant=Disabled  SatFdbkVariant=Disabled  DerivativeFilterVariant=ContFilter  NVariant=InternalParameters  NCopyVariant=Disabled  FilterICVariant=InternalICsFilter  IntegratorICVariant=InternalICs  ExternalResetVariant=Disabled  TRSumVariant=Passthrough  SumFdbkVariant=Disabled  SumVariant=Sum_PID
  Y PID Controller : simulink/Continuous/PID Controller  Controller=PID  Form=Parallel  TimeDomain=Continuous-time  SampleTime=-1  IntegratorMethod=Forward Euler  FilterMethod=Forward Euler  ControllerParametersSource=internal  P=86068.4824775323  I=1023.33964920396  D=873113.755595222  N=9.58373501278933  UseFilter=on  TunerSelectOption=Transfer Function Based (PID Tuner App)  InitialConditionSource=internal  InitialConditionForIntegrator=0  InitialConditionForFilter=0  DifferentiatorICPrevScaledInput=0  ExternalReset=none  TrackingMode=off  Kt=1  LimitOutput=off  UpperSaturationLimit=inf  LowerSaturationLimit=-inf  LinearizeAsGain=on  AntiWindupMode=none  Kb=1  POutMin=[]  POutMax=[]  IOutMin=[]  IOutMax=[]  DOutMin=[]  DOutMax=[]  NOutMin=[]  NOutMax=[]  SumOutMin=[]  SumOutMax=[]  SaturationOutMin=[]  SaturationOutMax=[]  PParamMin=[]  PParamMax=[]  IParamMin=[]  IParamMax=[]  DParamMin=[]  DParamMax=[]  NParamMin=[]  NParamMax=[]  KbParamMin=[]  KbParamMax=[]  KtParamMin=[]  KtParamMax=[]  KbOutMin=[]  KbOutMax=[]  KtOutMin=[]  KtOutMax=[]  IntegratorOutMin=[]  IntegratorOutMax=[]  FilterOutMin=[]  FilterOutMax=[]  SumI1OutMin=[]  SumI1OutMax=[]  SumI2OutMin=[]  SumI2OutMax=[]  SumI3OutMin=[]  SumI3OutMax=[]  SumI4OutMin=[]  SumI4OutMax=[]  SumDOutMin=[]  SumDOutMax=[]  DifferentiatorOutMin=[]  DifferentiatorOutMax=[]  FilterDiffOutCoefMin=[]  FilterDiffOutCoefMax=[]  ReciprocalOutMin=[]  ReciprocalOutMax=[]  SumDenOutMin=[]  SumDenOutMax=[]  SumNumOutMin=[]  SumNumOutMax=[]  DivideOutMin=[]  DivideOutMax=[]  IntegratorContinuousStateAttributes=''  IntegratorStateMustResolveToSignalObject=off  IntegratorRTWStateStorageClass=Auto  FilterContinuousStateAttributes=''  FilterStateMustResolveToSignalObject=off  FilterRTWStateStorageClass=Auto  ParallelPVariant=InternalParameters  IdealPVariant=Disabled  IVariant=InternalParameters  DVariant=InternalParameters  IntegratorVariant=Continuous  SatVariant=Disabled  AWVariant=Passthrough  PCopyVariant=Disabled  TRVariant=Disabled  FdbkBlocksVariant=Forward  IdealPFdbkVariant=Disabled  SatFdbkVariant=Disabled  DerivativeFilterVariant=ContFilter  NVariant=InternalParameters  NCopyVariant=Disabled  FilterICVariant=InternalICsFilter  IntegratorICVariant=InternalICs  ExternalResetVariant=Disabled  TRSumVariant=Passthrough  SumFdbkVariant=Disabled  SumVariant=Sum_PID
  Yaw PID Controller : simulink/Continuous/PID Controller  Controller=PID  Form=Parallel  TimeDomain=Continuous-time  SampleTime=-1  IntegratorMethod=Forward Euler  FilterMethod=Forward Euler  ControllerParametersSource=internal  P=22601532.1961172  I=216418.579552689  D=253682723.351677  N=0.143717056319525  UseFilter=on  TunerSelectOption=Transfer Function Based (PID Tuner App)  InitialConditionSource=internal  InitialConditionForIntegrator=0  InitialConditionForFilter=0  DifferentiatorICPrevScaledInput=0  ExternalReset=none  TrackingMode=off  Kt=1  LimitOutput=off  UpperSaturationLimit=inf  LowerSaturationLimit=-inf  LinearizeAsGain=on  AntiWindupMode=none  Kb=1  POutMin=[]  POutMax=[]  IOutMin=[]  IOutMax=[]  DOutMin=[]  DOutMax=[]  NOutMin=[]  NOutMax=[]  SumOutMin=[]  SumOutMax=[]  SaturationOutMin=[]  SaturationOutMax=[]  PParamMin=[]  PParamMax=[]  IParamMin=[]  IParamMax=[]  DParamMin=[]  DParamMax=[]  NParamMin=[]  NParamMax=[]  KbParamMin=[]  KbParamMax=[]  KtParamMin=[]  KtParamMax=[]  KbOutMin=[]  KbOutMax=[]  KtOutMin=[]  KtOutMax=[]  IntegratorOutMin=[]  IntegratorOutMax=[]  FilterOutMin=[]  FilterOutMax=[]  SumI1OutMin=[]  SumI1OutMax=[]  SumI2OutMin=[]  SumI2OutMax=[]  SumI3OutMin=[]  SumI3OutMax=[]  SumI4OutMin=[]  SumI4OutMax=[]  SumDOutMin=[]  SumDOutMax=[]  DifferentiatorOutMin=[]  DifferentiatorOutMax=[]  FilterDiffOutCoefMin=[]  FilterDiffOutCoefMax=[]  ReciprocalOutMin=[]  ReciprocalOutMax=[]  SumDenOutMin=[]  SumDenOutMax=[]  SumNumOutMin=[]  SumNumOutMax=[]  DivideOutMin=[]  DivideOutMax=[]  IntegratorContinuousStateAttributes=''  IntegratorStateMustResolveToSignalObject=off  IntegratorRTWStateStorageClass=Auto  FilterContinuousStateAttributes=''  FilterStateMustResolveToSignalObject=off  FilterRTWStateStorageClass=Auto  ParallelPVariant=InternalParameters  IdealPVariant=Disabled  IVariant=InternalParameters  DVariant=InternalParameters  IntegratorVariant=Continuous  SatVariant=Disabled  AWVariant=Passthrough  PCopyVariant=Disabled  TRVariant=Disabled  FdbkBlocksVariant=Forward  IdealPFdbkVariant=Disabled  SatFdbkVariant=Disabled  DerivativeFilterVariant=ContFilter  NVariant=InternalParameters  NCopyVariant=Disabled  FilterICVariant=InternalICsFilter  IntegratorICVariant=InternalICs  ExternalResetVariant=Disabled  TRSumVariant=Passthrough  SumFdbkVariant=Disabled  SumVariant=Sum_PID
  tau (body frame) : Outport  VectorParamsAs1DForOutWhenUnconnected=off
  wires:
  eta/1 -> Demux/1  "eta"
  eta set point/1 -> Demux1/1
  Demux/1 -> Sum2/1  "n_vessel"
  Demux1/1 -> Sum2/2  "n_sp"
  Demux/2 -> Sum/1  "e_vessel"
  Demux1/2 -> Sum/2  "e_sp"
  Sum2/1 -> Mux/1
  Sum/1 -> Mux/2
  MATLAB Function/1(y) -> Matrix Multiply/1
  Mux/1 -> Matrix Multiply/2  "error NED frame"
  Step/1 -> Mux2/4, Mux2/3, Mux2/5
  Demux1/3 -> Sum1/2, MATLAB Function1/1(u)  "yaw_sp"
  Sum1/1 -> Yaw PID Controller/1, Mux3/3
  Constant/1 -> Mux/3
  Demux/3 -> MATLAB Function/1(u), Sum1/1  "yaw_vessel"
  Matrix Multiply/1 -> Demux4/1  "error body frame"
  nu/1 -> Sum3/1
  Sum3/1 -> Gain/1  "error body frame"
  nu setpoint/1 -> Matrix Multiply1/2
  MATLAB Function1/1(y) -> Matrix Multiply1/1
  Matrix Multiply1/1 -> Sum3/2
  Integrator/1 -> Gain2/1
  Gain1/1 -> Add/1
  Gain2/1 -> Add/2
  Gain/1 -> Add/3
  Add/1 -> To Workspace/1, Scope/1, Manual Switch/2
  Demux3/1 -> Mux2/1
  Demux3/2 -> Mux2/2
  Demux3/3 -> Mux2/6
  Demux4/1 -> X PID Controller/1, Mux3/1
  Demux4/2 -> Y PID Controller/1, Mux3/2
  Demux4/3 -> Terminator1/1
  Mux3/1 -> Integrator/1, Gain1/1
  Mux2/1 -> tau (body frame)/1
  Manual Switch/1 -> Demux3/1
  X PID Controller/1 -> Mux1/1
  Y PID Controller/1 -> Mux1/2
  Yaw PID Controller/1 -> Mux1/3
  Mux1/1 -> Manual Switch/1

== system part2_MAIN_2019_for_ayon_because_he_cant_update_his_matlab/ Original/Observer ==
  y : Inport
  tau_est : Inport  Port=2
  Demux : Demux  Outputs=2
  EKF : Subsystem
  Memory : Memory  InitialCondition=zeros(3,1)
  Mux : Mux  Inputs=2
  Mux1 : Mux  Inputs=2
  Observer Selector : Constant  Value=observer_type
  Passive Non-Linear : Subsystem
  Subsystem : Subsystem
  Switch : Switch  Criteria=u2 > Threshold
  nu_hat : Outport  VectorParamsAs1DForOutWhenUnconnected=off
  eta_hat : Outport  Port=2  VectorParamsAs1DForOutWhenUnconnected=off
  wires:
  y/1 -> EKF/1(y), Passive Non-Linear/1(y)
  tau_est/1 -> Subsystem/1(In1)
  Memory/1 -> EKF/2(U)
  Subsystem/1(Out1) -> Memory/1, Passive Non-Linear/2(tau_est)
  EKF/1(eta_hat) -> Mux/1
  EKF/2(nu_hat) -> Mux/2
  Passive Non-Linear/1(eta_hat) -> Mux1/1
  Passive Non-Linear/2(nu_hat) -> Mux1/2
  Mux1/1 -> Switch/1
  Observer Selector/1 -> Switch/2
  Mux/1 -> Switch/3
  Switch/1 -> Demux/1
  Demux/1 -> eta_hat/1
  Demux/2 -> nu_hat/1

== system part2_MAIN_2019_for_ayon_because_he_cant_update_his_matlab/ Original/Reference Model ==
  note: Af
  note: eta_r
  note: Xref
  note: omega
  note: eta_r - Xref
  note: Gamma
  note: x_ddot
  note: Gamma
  note: X_dot
  note: X
  Add : Sum  Inputs=+--
  Gain : Gain  Gain=Af  Multiplication=Matrix(K*u)
  Gain1 : Gain  Gain=Gamma  Multiplication=Matrix(K*u)
  Gain2 : Gain  Gain=Omega  Multiplication=Matrix(K*u)
  Gain3 : Gain  Gain=Gamma  Multiplication=Matrix(K*u)
  Integrator : Integrator
  Integrator1 : Integrator
  Integrator2 : Integrator
  Scope : Scope  NumInputPorts=2
  Scope1 : Scope
  Scope2 : Scope
  Simulation Selector : Subsystem
  Sum : Sum  Inputs=|+-
  To Workspace : ToWorkspace  VariableName=Reference  SaveFormat=Timeseries  SampleTime=-1
  Set-point : Outport  VectorParamsAs1DForOutWhenUnconnected=off
  nu set point : Outport  Port=2  VectorParamsAs1DForOutWhenUnconnected=off
  wires:
  Integrator/1 -> Gain1/1, Sum/2
  Add/1 -> Scope2/1, Integrator1/1
  Integrator2/1 -> To Workspace/1, Scope/1, Set-point/1, Gain3/1
  Gain1/1 -> Add/1
  Integrator1/1 -> nu set point/1, Scope/2, Integrator2/1, Gain2/1
  Gain/1 -> Integrator/1
  Gain2/1 -> Add/3
  Gain3/1 -> Add/2
  Simulation Selector/1(Out1) -> Scope1/1, Sum/1
  Sum/1 -> Gain/1

== system part2_MAIN_2019_for_ayon_because_he_cant_update_his_matlab/ Original/Thrust Allocation ==
  tau_d : Inport
  MATLAB Function : MATLAB Function  TreatAsAtomicUnit=on
  MATLAB Function1 : MATLAB Function  Commented=on  TreatAsAtomicUnit=on
  MATLAB Function2 : MATLAB Function  Commented=on  TreatAsAtomicUnit=on
  MATLAB Function3 : MATLAB Function  Commented=on  TreatAsAtomicUnit=on
  Unwrap : Subsystem
  u : Outport  VectorParamsAs1DForOutWhenUnconnected=off
  alpha [rad] : Outport  Port=2  VectorParamsAs1DForOutWhenUnconnected=off
  wires:
  tau_d/1 -> MATLAB Function/1(tau_d), MATLAB Function1/1(tau_d)
  MATLAB Function1/1(Td) -> ?
  MATLAB Function1/2(alpha) -> ?
  MATLAB Function/1(Td) -> u/1
  MATLAB Function/2(alpha) -> Unwrap/1(alpha)
  Unwrap/1(alpha [rad]) -> alpha [rad]/1

== system part2_MAIN_2019_for_ayon_because_he_cant_update_his_matlab/ Original/Thruster Dynamics ==
  u [N] : Inport
  alpha [rad] : Inport  Port=2
  Constant : Constant  Value=[thrusters(1).xposition, thrusters(2).xposition, thrusters(3).xposition, thrusters(4).xposition, thrusters(5).xposition]
  Constant1 : Constant  Value=zeros(3,1)
  Constant2 : Constant  Value=[thrusters(1).yposition, thrusters(2).yposition, thrusters(3).yposition, thrusters(4).yposition, thrusters(5).yposition]
  Demux : Demux  Outputs=5
  Demux1 : Demux  Outputs=5
  Gain1 : Gain  Gain=1-thrusterfault
  Gain2 : Gain  Gain=1-thrusterfault
  MATLAB Function : MATLAB Function  TreatAsAtomicUnit=on
  Mux1 : Mux  Inputs=2
  Rate Limiter : RateLimiter  RisingSlewLimit=thrusters(1).rate  FallingSlewLimit=-thrusters(1).rate  SampleTimeMode=inherited
  Rate Limiter1 : RateLimiter  RisingSlewLimit=thrusters(2).rate  FallingSlewLimit=-thrusters(2).rate  SampleTimeMode=inherited
  Rate Limiter10 : RateLimiter  RisingSlewLimit=thrusters(4).rotationspeed  FallingSlewLimit=-thrusters(4).rotationspeed  SampleTimeMode=inherited
  Rate Limiter11 : RateLimiter  RisingSlewLimit=thrusters(5).rotationspeed  FallingSlewLimit=-thrusters(5).rotationspeed  SampleTimeMode=inherited
  Rate Limiter2 : RateLimiter  RisingSlewLimit=thrusters(3).rate  FallingSlewLimit=-thrusters(3).rate  SampleTimeMode=inherited
  Rate Limiter4 : RateLimiter  RisingSlewLimit=thrusters(4).rate  FallingSlewLimit=-thrusters(4).rate  SampleTimeMode=inherited
  Rate Limiter5 : RateLimiter  RisingSlewLimit=thrusters(5).rate  FallingSlewLimit=-thrusters(5).rate  SampleTimeMode=inherited
  Rate Limiter8 : RateLimiter  RisingSlewLimit=thrusters(2).rotationspeed  FallingSlewLimit=-thrusters(2).rotationspeed  SampleTimeMode=inherited
  Saturation : Saturate  UpperLimit=thrusters(1).thrust  LowerLimit=-thrusters(1).thrust
  Saturation1 : Saturate  UpperLimit=thrusters(2).thrust  LowerLimit=-thrusters(2).thrust
  Saturation2 : Saturate  UpperLimit=thrusters(3).thrust  LowerLimit=-thrusters(3).thrust
  Saturation4 : Saturate  UpperLimit=thrusters(4).thrust  LowerLimit=-thrusters(4).thrust
  Saturation5 : Saturate  UpperLimit=thrusters(5).thrust  LowerLimit=-thrusters(5).thrust
  Selector4 : Selector  InputPortWidth=6  IndexOptions=Index vector (dialog)  Indices=[1 2 4 5 6 3]  OutputSizes=1
  alpha : Mux  Inputs=5
  u : Mux  Inputs=5
  "Forces (body frame) " : Outport  VectorParamsAs1DForOutWhenUnconnected=off
  wires:
  Rate Limiter2/1 -> u/3
  Saturation/1 -> Rate Limiter/1
  Mux1/1 -> Selector4/1
  Constant1/1 -> Mux1/2
  Saturation4/1 -> Rate Limiter4/1
  Demux/2 -> Saturation1/1
  Saturation1/1 -> Rate Limiter1/1
  Demux/1 -> Saturation/1
  Demux/3 -> Saturation2/1
  Saturation2/1 -> Rate Limiter2/1
  Selector4/1 -> "Forces (body frame) "/1
  Gain1/1 -> u/2
  Rate Limiter1/1 -> Gain1/1
  Rate Limiter/1 -> u/1
  Rate Limiter4/1 -> Gain2/1
  Saturation5/1 -> Rate Limiter5/1
  u [N]/1 -> Demux/1
  alpha [rad]/1 -> Demux1/1
  Constant/1 -> MATLAB Function/3(PosX)
  Constant2/1 -> MATLAB Function/4(PosY)
  u/1 -> MATLAB Function/2(thrust_actual)
  alpha/1 -> MATLAB Function/1(alpha_actual)
  MATLAB Function/1(actual_tau) -> Mux1/1
  Rate Limiter10/1 -> alpha/4
  Demux1/4 -> Rate Limiter10/1
  Demux1/5 -> Rate Limiter11/1
  Rate Limiter11/1 -> alpha/5
  Demux1/1 -> alpha/1
  Gain2/1 -> u/4
  Demux/4 -> Saturation4/1
  Demux/5 -> Saturation5/1
  Rate Limiter5/1 -> u/5
  Demux1/2 -> Rate Limiter8/1
  Rate Limiter8/1 -> alpha/2
  Demux1/3 -> alpha/3

== system part2_MAIN_2019_for_ayon_because_he_cant_update_his_matlab/ Original/Wave ==
  eta : Inport
  waves : Inport  Port=2
  Gain : Gain  Gain=waveforces
  Sum : Sum
  Wave loads (U=0) : marine_hydro/Hydro Library/Wave loads (U=0)  SystemSampleTime=-1  Latency=0  AutoFrameSizeCalculation=off
  Wave : Outport  VectorParamsAs1DForOutWhenUnconnected=off
  wires:
  eta/1 -> Wave loads (U=0)/1
  waves/1 -> Wave loads (U=0)/2
  Sum/1 -> Gain/1
  Wave loads (U=0)/1 -> Sum/1
  Wave loads (U=0)/2 -> Sum/2
  Gain/1 -> Wave/1
